simulink model "PanelSolarSeguidor"  (R2022b)
settings: Solver=VariableStepAuto  StartTime=0.0  StopTime=10.0  RelTol=1e-3
model workspace (MAT data in the model file):
  Sig = Simulink.Signal
  Sig.DataType = 'auto'
  Sig.DocUnits = 'deg'
  Sig.Dimensions = -1
  Sig.DimensionsMode = 'auto'
  Sig.Complexity = 'auto'
  Sig.SampleTime = -1
  Sig.SamplingMode = 'auto'
values from neighbouring files (symbols this model uses):
  amplitude_sinewave = 10000    [PanelSolarSeguidor.mat]
  beta = 0.785398163397    [PanelSolarSeguidor.mat]    (also in PanelSolarSeguidor_3D.m = ans.logsout{2}.Values.Data)
  bias_sinewave = 0    [PanelSolarSeguidor.mat]
  constant = 1000    [PanelSolarSeguidor.mat]
  dph = 0.035    [PanelSolarSeguidor.mat]    (also in PanelSolarSeguidor_3D.m = 0.35)
  final_step = 4000    [PanelSolarSeguidor.mat]
  frec_sinewave = 1    [PanelSolarSeguidor.mat]
  initial_pendiente = 0    [PanelSolarSeguidor.mat]
  intial_step = 0    [PanelSolarSeguidor.mat]
  Kd = 5    [PanelSolarSeguidor.mat]    (also in PanelSolarSeguidor_3D.m)
  Kf = 1.835    [PanelSolarSeguidor.mat]    (also in PanelSolarSeguidor_3D.m)
  Kg = 20    [PanelSolarSeguidor.mat]    (also in PanelSolarSeguidor_3D.m)
  Kt = 1.835    [PanelSolarSeguidor.mat]    (also in PanelSolarSeguidor_3D.m)
  L = 0.1042    [PanelSolarSeguidor.mat]    (also in PanelSolarSeguidor_3D.m)
  m = 24.5    [PanelSolarSeguidor.mat]
  P_L = 2.18    [PanelSolarSeguidor_3D.m]
  P_W = 0.996    [PanelSolarSeguidor_3D.m]
  pendiente_rampa = 10000    [PanelSolarSeguidor.mat]
  phase_sinewave = 0    [PanelSolarSeguidor.mat]
  R = 3.05    [PanelSolarSeguidor.mat]    (also in PanelSolarSeguidor_3D.m)
  sampletime_sinewave = 0    [PanelSolarSeguidor.mat]
  sampletime_step = 2    [PanelSolarSeguidor.mat]
  selector = 4    [PanelSolarSeguidor.mat]
  steptime_step = 1    [PanelSolarSeguidor.mat]
libraries: simulink x4, simulink_extras x1
settings Model: Creator=marte  LastModifiedBy=marte

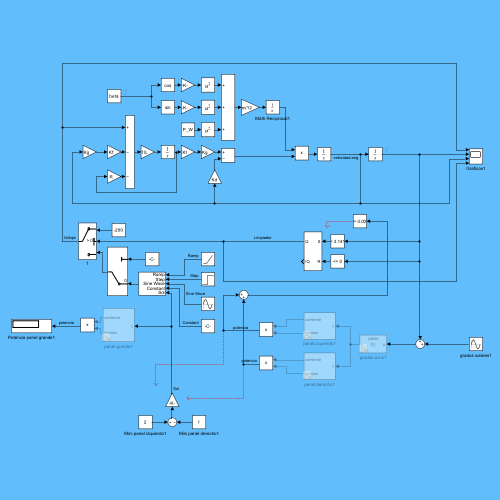
[thumbnail: Simulink's stored preview of the top-level diagram]
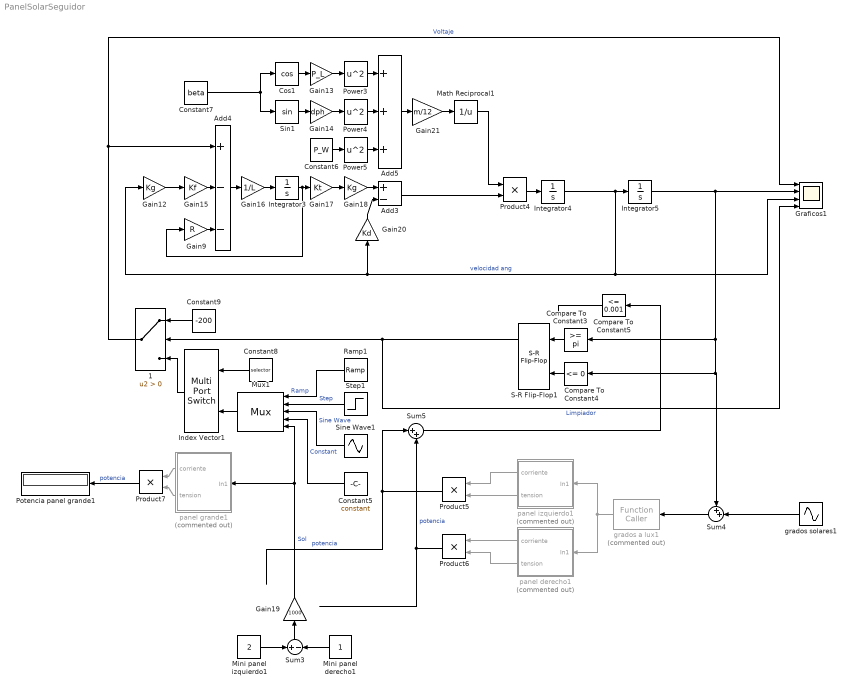
== system PanelSolarSeguidor ==
  1 : Switch  Criteria=u2 > Threshold  SaturateOnIntegerOverflow=off  InputSameDT=off
  Add3 : Sum  Inputs=+-
  Add4 : Sum  Inputs=+--
  Add5 : Sum  Inputs=+++
  Compare To Constant3 : simulink/Logic and Bit Operations/Compare To Constant  relop=>=  const=pi  OutDataTypeStr=boolean
  Compare To Constant4 : simulink/Logic and Bit Operations/Compare To Constant  relop=<=  const=0  OutDataTypeStr=boolean
  Compare To Constant5 : simulink/Logic and Bit Operations/Compare To Constant  relop=<=  const=0.001  OutDataTypeStr=boolean
  Constant5 : Constant  Value=constant
  Constant6 : Constant  Value=P_W
  Constant7 : Constant  Value=beta
  Constant8 : Constant  Value=selector
  Constant9 : Constant  Value=-200
  Cos1 : Trigonometry  Operator=cos
  Gain12 : Gain  Gain=Kg
  Gain13 : Gain  Gain=P_L
  Gain14 : Gain  Gain=dph
  Gain15 : Gain  Gain=Kf
  Gain16 : Gain  Gain=1/L
  Gain17 : Gain  Gain=Kt
  Gain18 : Gain  Gain=Kg
  Gain19 : Gain  Gain=1000
  Gain20 : Gain  Gain=Kd
  Gain21 : Gain  Gain=m/12
  Gain9 : Gain  Gain=R
  Graficos1 : Scope  NumInputPorts=4
  Index Vector1 : MultiPortSwitch  DataPortOrder=Zero-based contiguous  Inputs=1  zeroidx=on  SaturateOnIntegerOverflow=off  InputSameDT=off
  Integrator3 : Integrator
  Integrator4 : Integrator
  Integrator5 : Integrator
  Math Reciprocal1 : Math  Operator=reciprocal  SignedPower=on
  Mini panel derecho1 : Constant
  Mini panel izquierdo1 : Constant  Value=2
  Mux1 : Mux  Inputs=5
      settings: DisplayOption=signals
  Potencia panel grande1 : Display
  Power3 : Math  Operator=square
  Power4 : Math  Operator=square
  Power5 : Math  Operator=square
  Product{4..7} (4 alike) : Product
  Ramp1 : simulink/Sources/Ramp  slope=pendiente_rampa  start=start_time_pendiente  InitialOutput=initial_pendiente
  S-R Flip-Flop1 : simulink_extras/Flip Flops/S-R Flip-Flop  initial_condition=0
  Sin1 : Trigonometry
  Sine Wave1 : Sin  Amplitude=amplitude_sinewave  Bias=bias_sinewave  Frequency=frec_sinewave  Phase=phase_sinewave  SampleTime=sampletime_sinewave
  Step1 : Step  Time=steptime_step  Before=intial_step  After=final_step  SampleTime=sampletime_step
  Sum3 : Sum  Inputs=+|-
  Sum4 : Sum  Inputs=++|
  Sum5 : Sum  Inputs=|++
  grados a lux1 : FunctionCaller  Commented=on  FunctionPrototype=y = f(u)  InputArgumentSpecifications=<Enter example>  OutputArgumentSpecifications=<Enter example>
  grados solares1 : Sin  SampleTime=0
  panel derecho1 : Subsystem  Commented=on
  panel grande1 : Subsystem  Commented=on
  panel izquierdo1 : Subsystem  Commented=on
  wires:
  Compare To Constant5/1 -> ?
  grados solares1/1 -> Sum4/2
  Gain12/1 -> Gain15/1
  panel grande1/1(corriente) -> Product7/1
  panel grande1/2(tension) -> Product7/2
  Mini panel derecho1/1 -> Sum3/2
  Product5/1 -> Sum5/1  "potencia"
  Power5/1 -> Add5/3
  Product7/1 -> Potencia panel grande1/1  "potencia"
  Power3/1 -> Add5/1
  Sum5/1 -> Compare To Constant5/1
  Add5/1 -> Gain21/1
  Gain9/1 -> Add4/3
  panel derecho1/1(corriente) -> Product6/1
  Gain16/1 -> Integrator3/1
  panel izquierdo1/2(tension) -> Product5/2
  Compare To Constant3/1 -> S-R Flip-Flop1/1
  Product6/1 -> Sum5/2  "potencia"
  S-R Flip-Flop1/1 -> Graficos1/4, 1/2  "Limpiador"
  Step1/1 -> Mux1/2  "Step"
  panel derecho1/2(tension) -> Product6/2
  Gain19/1 -> Mux1/5, panel grande1/1(In1)  "Sol"
  1/1 -> Add4/1, Graficos1/1  "Voltaje"
  Gain15/1 -> Add4/2
  Product4/1 -> Integrator4/1
  Constant9/1 -> 1/1
  Constant8/1 -> Index Vector1/1
  Integrator5/1 -> Graficos1/2, Compare To Constant3/1, Compare To Constant4/1, Sum4/1
  Gain18/1 -> Add3/1
  Gain21/1 -> Math Reciprocal1/1
  Sin1/1 -> Gain14/1
  Ramp1/1 -> Mux1/1  "Ramp"
  Sine Wave1/1 -> Mux1/3  "Sine Wave"
  Math Reciprocal1/1 -> Product4/1
  Mux1/1 -> Index Vector1/2
  Sum4/1 -> grados a lux1/1
  Gain14/1 -> Power4/1
  Power4/1 -> Add5/2
  Cos1/1 -> Gain13/1
  Constant5/1 -> Mux1/4  "Constant"
  Mini panel izquierdo1/1 -> Sum3/1
  Add4/1 -> Gain16/1
  Add3/1 -> Product4/2
  Gain17/1 -> Gain18/1
  grados a lux1/1 -> panel izquierdo1/1(In1), panel derecho1/1(In1)
  Constant7/1 -> Cos1/1, Sin1/1
  Gain20/1 -> Add3/2
  panel izquierdo1/1(corriente) -> Product5/1
  Index Vector1/1 -> 1/3
  Integrator3/1 -> Gain17/1, Gain9/1
  Compare To Constant4/1 -> S-R Flip-Flop1/2
  Sum3/1 -> Gain19/1
  Constant6/1 -> Power5/1
  Gain13/1 -> Power3/1
  Integrator4/1 -> Integrator5/1, Gain20/1, Gain12/1, Graficos1/3  "velocidad ang"

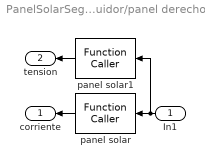
== system PanelSolarSeguidor/panel derecho1 ==
  In1 : Inport
  panel solar : FunctionCaller  FunctionPrototype=y = f(u)  InputArgumentSpecifications=<Enter example>  OutputArgumentSpecifications=<Enter example>
  panel solar1 : FunctionCaller  FunctionPrototype=y = f(u)  InputArgumentSpecifications=<Enter example>  OutputArgumentSpecifications=<Enter example>
  corriente : Outport
  tension : Outport  Port=2
  wires:
  In1/1 -> panel solar1/1, panel solar/1
  panel solar/1 -> corriente/1
  panel solar1/1 -> tension/1

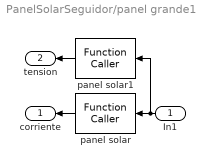
== system PanelSolarSeguidor/panel grande1 ==
  In1 : Inport
  panel solar : FunctionCaller  FunctionPrototype=y = f(u)  InputArgumentSpecifications=<Enter example>  OutputArgumentSpecifications=<Enter example>
  panel solar1 : FunctionCaller  FunctionPrototype=y = f(u)  InputArgumentSpecifications=<Enter example>  OutputArgumentSpecifications=<Enter example>
  corriente : Outport
  tension : Outport  Port=2
  wires:
  In1/1 -> panel solar1/1, panel solar/1
  panel solar/1 -> corriente/1
  panel solar1/1 -> tension/1

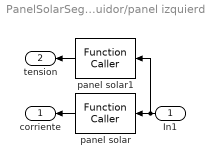
== system PanelSolarSeguidor/panel izquierdo1 ==
  In1 : Inport
  panel solar : FunctionCaller  FunctionPrototype=y = f(u)  InputArgumentSpecifications=<Enter example>  OutputArgumentSpecifications=<Enter example>
  panel solar1 : FunctionCaller  FunctionPrototype=y = f(u)  InputArgumentSpecifications=<Enter example>  OutputArgumentSpecifications=<Enter example>
  corriente : Outport
  tension : Outport  Port=2
  wires:
  In1/1 -> panel solar1/1, panel solar/1
  panel solar/1 -> corriente/1
  panel solar1/1 -> tension/1
